simulink model "Bai05"  (R2023b)
settings: Solver=VariableStepAuto  StartTime=0.0  StopTime=0.1  RelTol=1e-3
settings Model: Creator=Trung  LastModifiedBy=Trung

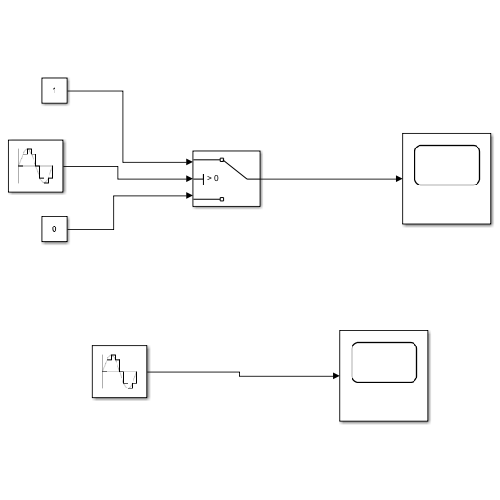
[thumbnail: Simulink's stored preview of the top-level diagram]
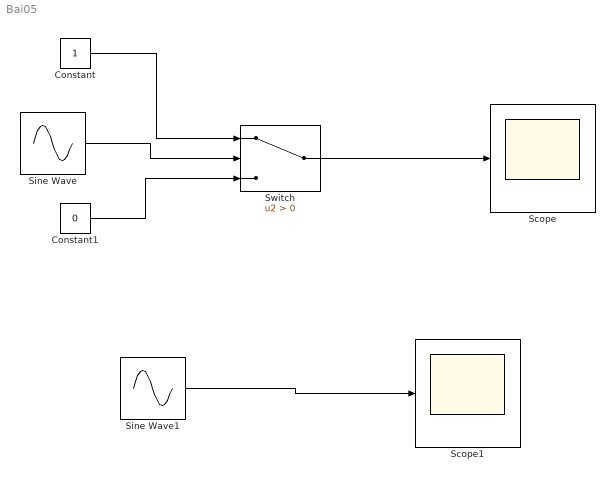
== system Bai05 ==
  Constant : Constant
  Constant1 : Constant  Value=0
  Scope : Scope
  Scope1 : Scope
  Sine Wave : Sin  Frequency=50 * pi * 2  Phase=pi  SampleTime=0.0001
  Sine Wave1 : Sin  Frequency=50 * pi * 2  Phase=pi  SampleTime=0.0001
  Switch : Switch  Criteria=u2 > Threshold  SaturateOnIntegerOverflow=off  InputSameDT=off
  wires:
  Constant/1 -> Switch/1
  Constant1/1 -> Switch/3
  Switch/1 -> Scope/1
  Sine Wave/1 -> Switch/2
  Sine Wave1/1 -> Scope1/1
